simulink model "IdealGen_load_CtrlGen_wDC_abc"  (R2023b)
settings: Solver=VariableStepAuto  StartTime=0.0  StopTime=12  RelTol=1e-3
undefined symbols (not defined in the file): C_dc, H_vsm, I_dc_0, I_dc_base, Ibase_lv, k_d_vsm, k_p_p_vsm, k_p_q_vsm, ki_q, l_f, L_grid, Lbase1v, omega_nom, Pmax, r_f, R_grid, Sbase1, Tchange_gfm_ref, Ts, V_dc, V_dc_base, Vbase_lv, Zbase1v
libraries: spsControlledVoltageSourceLib x6, spsThreePhaseVIMeasurementLib x3, spsPower3phInstantaneousLib x3, spsRMSLib x3, spsdq0toabcLib x2, spsCurrentMeasurementLib x2, spsDCVoltageSourceLib x2, spsSeriesRLCBranchLib x2, spsVoltageMeasurementLib x2, slpidlib x2, spsThreePhaseSeriesRLCBranchLib x2, spsGroundLib x1
settings Model: Creator=s183702  LastModifiedBy=marti

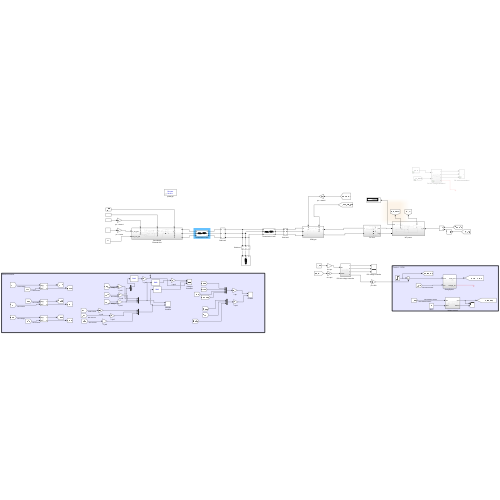
[thumbnail: Simulink's stored preview of the top-level diagram]
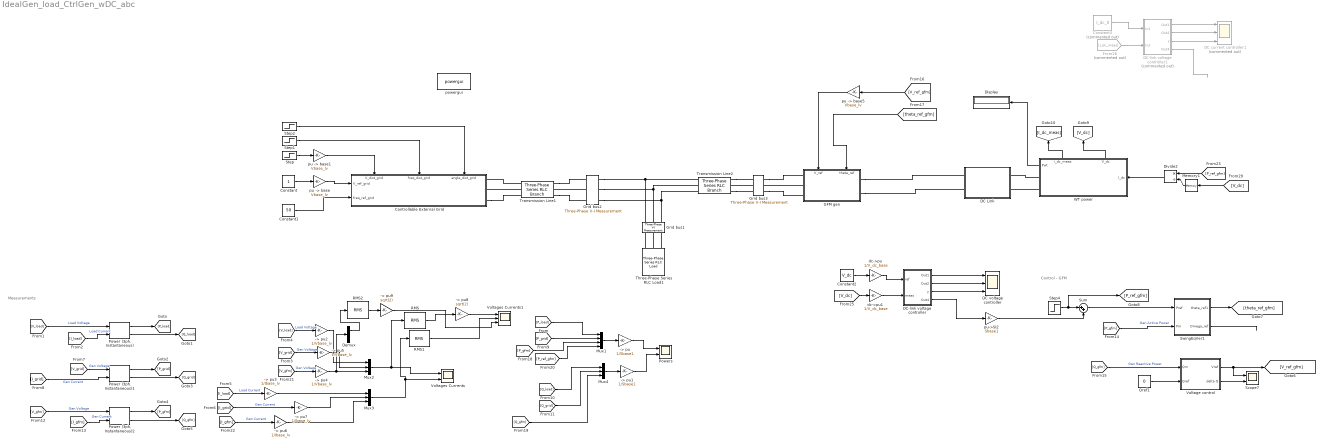
== system IdealGen_load_CtrlGen_wDC_abc ==
  note: Control - GFM
  note: Measurements
  -> pu : Gain  Gain=1/Sbase1
  -> pu1 : Gain  Gain=1/Sbase1
  -> pu2 : Gain  Gain=1/Vbase_lv
  -> pu3 : Gain  Gain=1/Ibase_lv
  -> pu4 : Gain  Gain=1/Vbase_lv
  -> pu5 : Gain  Gain=1/Vbase_lv
  -> pu6 : Gain  Gain=1/Ibase_lv
  -> pu7 : Gain  Gain=1/Ibase_lv
  -> pu8 : Gain  Gain=sqrt(2)
  -> pu9 : Gain  Gain=sqrt(2)
  Constant : Constant
  Constant1 : Constant  Value=50
  Constant2 : Constant  Value=V_dc
  Constant3 : Constant  Commented=on  Value=I_dc_0
  Controllable External Grid : Subsystem
      settings: PortSchema="{\"entries\":[{\"content\":{\"sides\":[{\"content\":{\"connectorIds\":[\"In1\",\"In2\"]},\"type\":\"ConnectorPlacement.EquallySpacedRectSide\",\"uuid\":\"c82e3ee4-47de-4631-9682-a189e406d2fd\"},{\"content\":{\"connectorIds\":[\"RConn1\",\"RConn2\",\"RConn3\"],\"side\":\"RIGHT\"},\"type\":\"ConnectorPlacement.EquallySpacedRectSide\",\"uuid\":\"b806e225-811d-4112-8c3d-45e9b8086e84\"},{\"content\":{\"connectorIds\":[\"In3\",\"In4\",\"In5\"],\"side\":\"TOP\"},\"type\":\"ConnectorPlacement.EquallySpacedRectSide\",\"uuid\":\"c79b677b-bc74-4454-b0f0-10f0f27e0767\"}]},\"type\":\"ConnectorPlacement.EquallySpacedConnector\",\"uuid\":\"44354c03-b4f0-403a-803b-b669dc1296a6\"}],\"packageUris\":[\"http://schema.mathworks.com/mf0/Connector/R2020b\"],\"version\":\"1.0\"}"
  DC Link : Subsystem
  DC current controller1 : Scope  Commented=on  NumInputPorts=3
  DC voltage controller : Scope  NumInputPorts=3
  DC-link voltage controller : Subsystem
  DC-link voltage controller1 : Subsystem  Commented=on
  Demux : Demux  Outputs=3
  Display : Display
  Divide2 : Product  Inputs=*/
  From26 : From  Commented=on  GotoTag=I_dc_meas
  GFM gen : Subsystem
      settings: PortSchema="{\"entries\":[{\"content\":{\"sides\":[{\"content\":{\"connectorIds\":[\"LConn1\",\"LConn2\"]},\"type\":\"ConnectorPlacement.EquallySpacedRectSide\",\"uuid\":\"b9b898d8-aa2c-4fc0-879f-33950e845205\"},{\"content\":{\"connectorIds\":[\"RConn1\",\"RConn2\",\"RConn3\"],\"side\":\"RIGHT\"},\"type\":\"ConnectorPlacement.EquallySpacedRectSide\",\"uuid\":\"0f5f2870-ceda-40eb-961f-274893a00dd5\"},{\"content\":{\"connectorIds\":[\"In1\",\"In2\"],\"side\":\"TOP\"},\"type\":\"ConnectorPlacement.EquallySpacedRectSide\",\"uuid\":\"16b0f3cd-2bcf-4c98-bcc9-1e9131637ccf\"}]},\"type\":\"ConnectorPlacement.EquallySpacedConnector\",\"uuid\":\"5f5ec50b-7fca-4ced-b434-e49ba9676af4\"}],\"packageUris\":[\"http://schema.mathworks.com/mf0/Connector/R2020b\"],\"version\":\"1.0\"}"
  Grid bus1 : spsThreePhaseVIMeasurementLib/Three-Phase V-I Measurement  VoltageMeasurement=phase-to-ground  SetLabelV=on  LabelV=V_load  Vpu=off  VpuLL=off  CurrentMeasurement=yes  SetLabelI=on  LabelI=I_load  Ipu=off  Pbase=100e6  Vbase=500e3  OutputType=Complex  PhasorSimulation=off  PSBequivalent=0
  Grid bus2 : spsThreePhaseVIMeasurementLib/Three-Phase V-I Measurement  VoltageMeasurement=phase-to-ground  SetLabelV=on  LabelV=V_grid  Vpu=off  VpuLL=off  CurrentMeasurement=yes  SetLabelI=on  LabelI=I_grid  Ipu=off  Pbase=100e6  Vbase=500e3  OutputType=Complex  PhasorSimulation=off  PSBequivalent=0
  Grid bus3 : spsThreePhaseVIMeasurementLib/Three-Phase V-I Measurement  VoltageMeasurement=phase-to-ground  SetLabelV=on  LabelV=V_gfm  Vpu=off  VpuLL=off  CurrentMeasurement=yes  SetLabelI=on  LabelI=I_gfm  Ipu=off  Pbase=100e6  Vbase=500e3  OutputType=Complex  PhasorSimulation=off  PSBequivalent=0
  Memory1 : Memory  InitialCondition=V_dc
  Mux1 : Mux
  Mux2 : Mux  Inputs=3
  Mux3 : Mux  Inputs=3
  Mux4 : Mux  Inputs=3
  "Power (3ph, Instantaneous)" : spsPower3phInstantaneousLib/Power (3ph, Instantaneous)
  "Power (3ph, Instantaneous)1" : spsPower3phInstantaneousLib/Power (3ph, Instantaneous)
  "Power (3ph, Instantaneous)2" : spsPower3phInstantaneousLib/Power (3ph, Instantaneous)
  Powers : Scope  NumInputPorts=2
  Qref1 : Constant  Value=0
  RMS : spsRMSLib/RMS  TrueRMS=on  Freq=50  RMSInit=1  Ts=0
  RMS1 : spsRMSLib/RMS  TrueRMS=on  Freq=50  RMSInit=1  Ts=0
  RMS2 : spsRMSLib/RMS  TrueRMS=on  Freq=50  RMSInit=1  Ts=0
  Scope7 : Scope  NumInputPorts=2
  Step : Step  After=0  SampleTime=0
  Step1 : Step  After=0  SampleTime=0
  Step2 : Step  After=0  SampleTime=0
  Step4 : Step  Time=Tchange_gfm_ref  Before=Sbase1  After=Sbase1  SampleTime=0
  Sum : Sum  Inputs=|++
  SwingEqVer1 : Subsystem
  Three-Phase Series RLC Load1 : spsThreePhaseSeriesRLCLoadLib/Three-Phase Series RLC Load  LConnTagsString=A|B|C  Configuration=Y (grounded)  NominalVoltage=Vbase_lv*sqrt(3/2)  Vabc=[1e3 1e3 1e3]  Vabcp=[1e3 1e3 1e3]  NominalFrequency=f_nom  UnbalancedPower=off  ActivePower=Sbase1*0.2  InductivePower=0  CapacitivePower=0  Pabc=[10e3 9e3 11e3]  QLabc=[100 90 110]  QCabc=[100 90 110]  Pabcp=[10e3 9e3 11e3]  QLabcp=[100 90 110]  QCabcp=[100 90 110]  Measurements=None  LoadType=constant PQ
  Transmission Line1 : spsThreePhaseSeriesRLCBranchLib/Three-Phase Series RLC Branch  LConnTagsString=A|B|C  RConnTagsString=A|B|C  BranchType=RL  Resistance=R_grid  Inductance=L_grid  Capacitance=0  Measurements=None
  Transmission Line2 : spsThreePhaseSeriesRLCBranchLib/Three-Phase Series RLC Branch  LConnTagsString=A|B|C  RConnTagsString=A|B|C  BranchType=RL  Resistance=r_f*Zbase1v  Inductance=l_f*Lbase1v  Capacitance=0  Measurements=None
  Voltage control : Subsystem
  Voltages Currents : Scope  NumInputPorts=2
  Voltages Currents1 : Scope  NumInputPorts=3
  WT power : Subsystem
      settings: PortSchema="{\"entries\":[{\"content\":{\"sides\":[{\"content\":{\"connectorIds\":[\"In1\"]},\"type\":\"ConnectorPlacement.EquallySpacedRectSide\",\"uuid\":\"9d3e38d2-6add-483d-9a31-3b5598dff8d3\"},{\"content\":{\"connectorIds\":[\"Out1\",\"RConn1\",\"RConn2\"],\"side\":\"RIGHT\"},\"type\":\"ConnectorPlacement.EquallySpacedRectSide\",\"uuid\":\"7ce5d226-07b0-4d85-bacd-eba224635451\"},{\"content\":{\"connectorIds\":[\"Out2\",\"Out3\"],\"side\":\"TOP\"},\"type\":\"ConnectorPlacement.EquallySpacedRectSide\",\"uuid\":\"1864accd-580c-4e01-b41e-4bc1921d0b77\"},{\"content\":{\"side\":\"BOTTOM\"},\"type\":\"ConnectorPlacement.EquallySpacedRectSide\",\"uuid\":\"0a771f6d-f5fb-412d-b2d7-9d95c39f39de\"}]},\"type\":\"ConnectorPlacement.EquallySpacedConnector\",\"uuid\":\"874bd654-abb7-47d1-80fe-1eaf36f4fe8a\"}],\"packageUris\":[\"http://schema.mathworks.com/mf0/Connector/R2020b\"],\"version\":\"1.0\"}"
  dc->pu : Gain  Gain=1/V_dc_base
  dc->pu1 : Gain  Gain=1/V_dc_base
  powergui : sps_lib/powergui  Priority=1  SimulationMode=Discrete  SampleTime=Ts  frequency=60  Iterations=50  frequencyindice=0  Pbase=100e6  ErrMax=1e-4  UnitsV=kV  UnitsW=MW  buscounter=0  FunctionMessages=off  echomessages=off  EnableUseOfTLC=off  CurrentSourceSwitches=off  DisableSnubberDevices=off  DisableRonSwitches=off  DisableVfSwitches=off  DisplayEquations=off  AutomaticDiscreteSolvers=off  SolverType=Tustin/Backward Euler (TBE)  Interpol=off  ExternalGateDelay=off  methode=off  Ts=100  x0status=blocks  SPID=on  SwTol=0  HookPort=off  NonlinearTolerance=1e-4  nMaxIteration=100  ContinueOnMaxIteration=off  RestoreLinks=warning  ResistiveCurrentMeasurement=off  Frange=[0:2:500]  Ylog=off  Xlog=on  ShowGrid=off  save=off  variable=ZData  structure=0  ZoomFFT=off  StartTime=0.0  cycles=1  DisplayStyle=1  fundamental=60  FreqAxis=off  MaxFrequency=1000  frequencyindicesteady=1  RmsSteady=1  display=off
  "pu -> base" : Gain  Gain=Vbase_lv
  "pu -> base1" : Gain  Gain=Vbase_lv
  "pu -> base5" : Gain  Gain=Vbase_lv
  pu->SI2 : Gain  Gain=Sbase1
  wires:
  [I_load] -> -> pu3/1  "Load Current"
  [V_load] -> -> pu2/1  "Load Voltage"
  [V_grid] -> -> pu5/1  "Gen Voltage"
  [I_grid] -> -> pu7/1  "Gen Current"
  "pu -> base"/1 -> Controllable External Grid/1(V_ref_grid)
  Constant/1 -> "pu -> base"/1
  Constant1/1 -> Controllable External Grid/2(freq_ref_grid)
  Step/1 -> "pu -> base1"/1
  Step1/1 -> Controllable External Grid/4(freq_dist_grid)
  Step2/1 -> Controllable External Grid/5(angle_dist_grid)
  "pu -> base1"/1 -> Controllable External Grid/3(V_dist_grid)
  [V_load] -> "Power (3ph, Instantaneous)"/1  "Load Voltage"
  [I_load] -> "Power (3ph, Instantaneous)"/2  "Load Current"
  [V_grid] -> "Power (3ph, Instantaneous)1"/1  "Gen Voltage"
  [I_grid] -> "Power (3ph, Instantaneous)1"/2  "Gen Current"
  "Power (3ph, Instantaneous)"/1 -> [P_load]
  "Power (3ph, Instantaneous)"/2 -> [Q_load]
  "Power (3ph, Instantaneous)1"/1 -> [P_grid]
  "Power (3ph, Instantaneous)1"/2 -> [Q_grid]
  [Q_load] -> Mux4/1
  [Q_grid] -> Mux4/2
  [P_grid] -> Mux1/2
  [P_load] -> Mux1/1
  Mux4/1 -> -> pu1/1
  Mux1/1 -> -> pu/1
  -> pu/1 -> Powers/1
  -> pu1/1 -> Powers/2
  "pu -> base5"/1 -> GFM gen/2(V_ref)
  "Power (3ph, Instantaneous)2"/2 -> [Q_gfm]
  "Power (3ph, Instantaneous)2"/1 -> [P_gfm]
  [I_gfm] -> "Power (3ph, Instantaneous)2"/2  "Gen Current"
  [V_gfm] -> "Power (3ph, Instantaneous)2"/1  "Gen Voltage"
  Sum/1 -> SwingEqVer1/1(Pref)
  [P_gfm] -> SwingEqVer1/2(Pm)  "Gen Active Power"
  SwingEqVer1/2(Omega_ref) -> ?
  SwingEqVer1/1(theta_ref1) -> [theta_ref_gfm]
  Qref1/1 -> Voltage control/2(Qref)
  Voltage control/1(Vref) -> Scope7/1, [V_ref_gfm]
  Voltage control/2(delta Q) -> Scope7/2
  [Q_gfm] -> Voltage control/1(Qm)  "Gen Reactive Power"
  [V_ref_gfm] -> "pu -> base5"/1
  [theta_ref_gfm] -> GFM gen/1(theta_ref)
  [P_gfm] -> Mux1/3
  [Q_gfm] -> Mux4/3
  [P_ref_gfm] -> Mux1/4
  [V_gfm] -> -> pu4/1  "Gen Voltage"
  [I_gfm] -> -> pu6/1  "Gen Current"
  Mux2/1 -> RMS/1, Voltages Currents/1
  Mux3/1 -> RMS1/1, Voltages Currents/2
  -> pu2/1 -> Mux2/1
  -> pu4/1 -> Demux/1, Mux2/3
  -> pu5/1 -> Mux2/2
  -> pu3/1 -> Mux3/1
  -> pu6/1 -> Mux3/3
  RMS/1 -> -> pu8/1
  RMS1/1 -> Voltages Currents1/2
  -> pu7/1 -> Mux3/2
  -> pu8/1 -> Voltages Currents1/1
  RMS2/1 -> -> pu9/1
  -> pu9/1 -> Voltages Currents1/3
  Demux/1 -> RMS2/1
  WT power/2(V_dc) -> [V_dc]
  WT power/1(Pwt) -> Display/1
  DC-link voltage controller1/4(Out4) -> ?
  Constant2/1 -> dc->pu/1
  [V_dc] -> dc->pu1/1
  DC-link voltage controller/1(Out1) -> DC voltage controller/1
  DC-link voltage controller/2(Out2) -> DC voltage controller/2
  DC-link voltage controller/3(y) -> DC voltage controller/3
  WT power/3(i_dc_meas) -> [I_dc_meas]
  From26/1 -> DC-link voltage controller1/2(In2)
  Constant3/1 -> DC-link voltage controller1/1(In1)
  DC-link voltage controller1/1(Out1) -> DC current controller1/1
  DC-link voltage controller1/2(Out2) -> DC current controller1/2
  DC-link voltage controller1/3(y) -> DC current controller1/3
  [P_ref_gfm] -> Divide2/1
  [V_dc] -> Memory1/1
  Memory1/1 -> Divide2/2
  Divide2/1 -> WT power/1(I_dc)
  dc->pu/1 -> DC-link voltage controller/1(ref)
  dc->pu1/1 -> DC-link voltage controller/2(meas)
  DC-link voltage controller/4(Out4) -> pu->SI2/1
  Step4/1 -> [P_ref_gfm], Sum/1
  pu->SI2/1 -> Sum/2
  connections:
  Three-Phase Series RLC Load1/LConn1 -- Grid bus1/RConn1
  Three-Phase Series RLC Load1/LConn2 -- Grid bus1/RConn2
  Three-Phase Series RLC Load1/LConn3 -- Grid bus1/RConn3
  Transmission Line2/LConn2 -- Grid bus2/RConn2 -- Grid bus1/LConn2
  Grid bus1/LConn1 -- Transmission Line2/LConn1 -- Grid bus2/RConn1
  Grid bus1/LConn3 -- Transmission Line2/LConn3 -- Grid bus2/RConn3
  Transmission Line1/RConn1 -- Grid bus2/LConn1
  Grid bus2/LConn2 -- Transmission Line1/RConn2
  Transmission Line1/RConn3 -- Grid bus2/LConn3
  Transmission Line1/LConn1 -- Controllable External Grid/RConn1
  Transmission Line1/LConn2 -- Controllable External Grid/RConn2
  Controllable External Grid/RConn3 -- Transmission Line1/LConn3
  GFM gen/RConn2 -- Grid bus3/LConn2
  Grid bus3/LConn1 -- GFM gen/RConn1
  Grid bus3/LConn3 -- GFM gen/RConn3
  Transmission Line2/RConn1 -- Grid bus3/RConn1
  Grid bus3/RConn2 -- Transmission Line2/RConn2
  Transmission Line2/RConn3 -- Grid bus3/RConn3
  GFM gen/LConn2 -- DC Link/LConn2
  GFM gen/LConn1 -- DC Link/LConn1
  WT power/RConn1 -- DC Link/RConn1
  WT power/RConn2 -- DC Link/RConn2

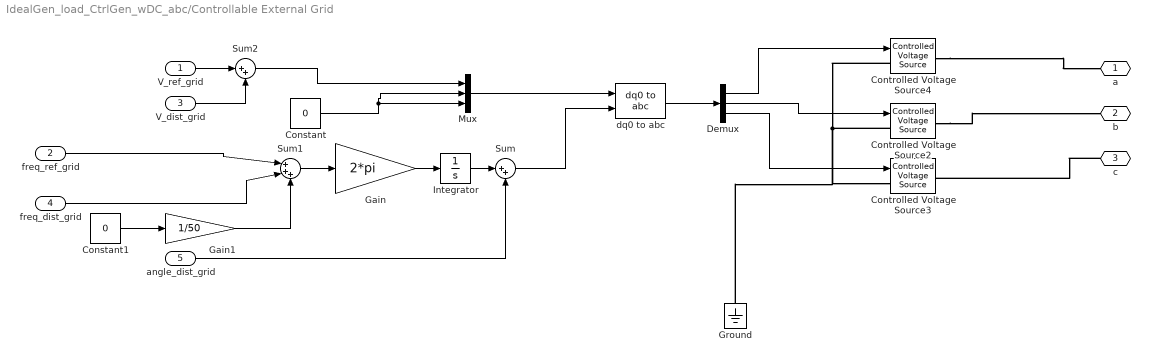
== system IdealGen_load_CtrlGen_wDC_abc/Controllable External Grid ==
  V_ref_grid : Inport
  freq_ref_grid : Inport  Port=2
  V_dist_grid : Inport  Port=3
  freq_dist_grid : Inport  Port=4
  angle_dist_grid : Inport  Port=5
  Constant : Constant  Value=0
  Constant1 : Constant  Value=0
  Controlled Voltage Source2 : spsControlledVoltageSourceLib/Controlled Voltage Source  Initialize=on  Source_Type=AC  Amplitude=Vbase_lv  Phase=-120  Frequency=50  Measurements=None
  Controlled Voltage Source3 : spsControlledVoltageSourceLib/Controlled Voltage Source  Initialize=on  Source_Type=AC  Amplitude=Vbase_lv  Phase=120  Frequency=50  Measurements=None
  Controlled Voltage Source4 : spsControlledVoltageSourceLib/Controlled Voltage Source  Initialize=on  Source_Type=AC  Amplitude=Vbase_lv  Phase=0  Frequency=50  Measurements=None
  Demux : Demux  Outputs=3
  Gain : Gain  Gain=2*pi
  Gain1 : Gain  Gain=1/50
  Ground : spsGroundLib/Ground  LConnTagsString=a
  Integrator : Integrator
  Mux : Mux  Inputs=3
  Sum : Sum  Inputs=|++
  Sum1 : Sum  Inputs=|+++
  Sum2 : Sum  Inputs=|++
  dq0 to abc : spsdq0toabcLib/dq0 to abc  Alignment=Aligned with phase A axis
  a : PMIOPort  Side=Right
  b : PMIOPort  Port=2  Side=Right
  c : PMIOPort  Port=3  Side=Right
  wires:
  Demux/1 -> Controlled Voltage Source4/1
  Demux/2 -> Controlled Voltage Source2/1
  Demux/3 -> Controlled Voltage Source3/1
  Mux/1 -> dq0 to abc/1
  Constant/1 -> Mux/2, Mux/3
  dq0 to abc/1 -> Demux/1
  Sum2/1 -> Mux/1
  Gain/1 -> Integrator/1
  Integrator/1 -> Sum/1
  angle_dist_grid/1 -> Sum/2
  freq_dist_grid/1 -> Sum1/2
  Sum1/1 -> Gain/1
  freq_ref_grid/1 -> Sum1/1
  Sum/1 -> dq0 to abc/2
  V_ref_grid/1 -> Sum2/1
  V_dist_grid/1 -> Sum2/2
  Gain1/1 -> Sum1/3
  Constant1/1 -> Gain1/1
  connections:
  Controlled Voltage Source2/LConn1 -- Controlled Voltage Source4/LConn1 -- Ground/LConn1 -- Controlled Voltage Source3/LConn1
  c/RConn1 -- Controlled Voltage Source3/RConn1
  Controlled Voltage Source4/RConn1 -- a/RConn1
  Controlled Voltage Source2/RConn1 -- b/RConn1

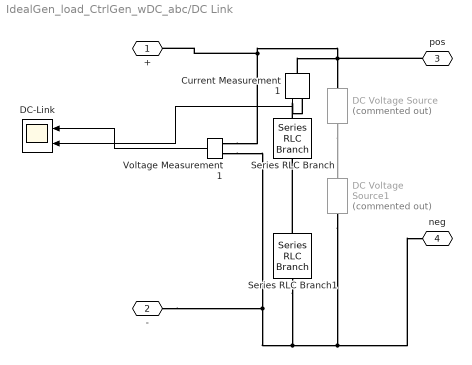
== system IdealGen_load_CtrlGen_wDC_abc/DC Link ==
  Current Measurement1 : spsCurrentMeasurementLib/Current Measurement  PhasorSimulation=off  OutputType=Complex  PSBequivalent=0
  DC Voltage Source : spsDCVoltageSourceLib/DC Voltage Source  Commented=on  Amplitude=V_dc/2  Measurements=None
  DC Voltage Source1 : spsDCVoltageSourceLib/DC Voltage Source  Commented=on  Amplitude=V_dc/2  Measurements=None
  DC-Link : Scope  NumInputPorts=2
  Series RLC Branch : spsSeriesRLCBranchLib/Series RLC Branch  LConnTagsString=__new0  RConnTagsString=__new0  BranchType=C  Resistance=1  Inductance=1e-3  SetiL0=off  InitialCurrent=0  Capacitance=C_dc/2  Setx0=on  InitialVoltage=V_dc/2  Measurements=None
  Series RLC Branch1 : spsSeriesRLCBranchLib/Series RLC Branch  LConnTagsString=__new0  RConnTagsString=__new0  BranchType=C  Resistance=1  Inductance=1e-3  SetiL0=off  InitialCurrent=0  Capacitance=C_dc/2  Setx0=on  InitialVoltage=V_dc/2  Measurements=None
  Voltage Measurement1 : spsVoltageMeasurementLib/Voltage Measurement  PhasorSimulation=off  OutputType=Complex  PSBequivalent=0
  + : PMIOPort  Side=Left
  - : PMIOPort  Port=2  Side=Left
  pos : PMIOPort  Port=3  Side=Right
  neg : PMIOPort  Port=4  Side=Right
  wires:
  Voltage Measurement1/1 -> DC-Link/1
  Current Measurement1/1 -> DC-Link/2
  connections:
  DC Voltage Source/LConn1 -- DC Voltage Source1/RConn1
  -/RConn1 -- Series RLC Branch1/RConn1 -- DC Voltage Source1/LConn1 -- neg/RConn1 -- Voltage Measurement1/LConn2
  Series RLC Branch1/LConn1 -- Series RLC Branch/RConn1
  pos/RConn1 -- Current Measurement1/LConn1 -- +/RConn1 -- Voltage Measurement1/LConn1 -- DC Voltage Source/RConn1
  Series RLC Branch/LConn1 -- Current Measurement1/RConn1

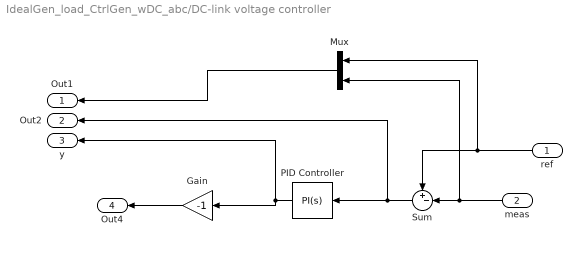
== system IdealGen_load_CtrlGen_wDC_abc/DC-link voltage controller ==
  ref : Inport
  meas : Inport  Port=2
  Gain : Gain  Gain=-1
  Mux : Mux  Inputs=2
  PID Controller : slpidlib/PID Controller  Controller=PI  Form=Parallel  TimeDomain=Continuous-time  UseExternalTs=off  SampleTime=-1  IntegratorMethod=Forward Euler  FilterMethod=Forward Euler  ControllerParametersSource=internal  P=5  I=1  UseKiTs=off  D=0  N=100  UseFilter=on  TunerSelectOption=Transfer Function Based (PID Tuner App)  InitialConditionSource=internal  InitialConditionForIntegrator=0  InitialConditionForFilter=0  DifferentiatorICPrevScaledInput=0  ExternalReset=none  TrackingMode=off  Kt=1  LimitOutput=off  SatLimitsSource=internal  UpperSaturationLimit=inf  LowerSaturationLimit=-inf  LinearizeAsGain=on  AntiWindupMode=none  Kb=1  LimitIntegrator=off  UpperIntegratorSaturationLimit=inf  LowerIntegratorSaturationLimit=-inf  POutMin=[]  POutMax=[]  IOutMin=[]  IOutMax=[]  DOutMin=[]  DOutMax=[]  NOutMin=[]  NOutMax=[]  SumOutMin=[]  SumOutMax=[]  SaturationOutMin=[]  SaturationOutMax=[]  PParamMin=[]  PParamMax=[]  IParamMin=[]  IParamMax=[]  DParamMin=[]  DParamMax=[]  NParamMin=[]  NParamMax=[]  KbParamMin=[]  KbParamMax=[]  KtParamMin=[]  KtParamMax=[]  KbOutMin=[]  KbOutMax=[]  KtOutMin=[]  KtOutMax=[]  IntegratorOutMin=[]  IntegratorOutMax=[]  FilterOutMin=[]  FilterOutMax=[]  SumI1OutMin=[]  SumI1OutMax=[]  SumI2OutMin=[]  SumI2OutMax=[]  SumI3OutMin=[]  SumI3OutMax=[]  SumI4OutMin=[]  SumI4OutMax=[]  SumDOutMin=[]  SumDOutMax=[]  DifferentiatorOutMin=[]  DifferentiatorOutMax=[]  FilterDiffOutCoefMin=[]  FilterDiffOutCoefMax=[]  ReciprocalOutMin=[]  ReciprocalOutMax=[]  SumDenOutMin=[]  SumDenOutMax=[]  SumNumOutMin=[]  SumNumOutMax=[]  DivideOutMin=[]  DivideOutMax=[]  UdiffTsProdOutMin=[]  UdiffTsProdOutMax=[]  NTsProdOutMin=[]  NTsProdOutMax=[]  UintegralTsProdOutMin=[]  UintegralTsProdOutMax=[]  UngainTsProdOutMin=[]  UngainTsProdOutMax=[]  ClampingZeroOutDataTypeStr=Inherit: Inherit via back propagation  ClampingZeroOutMin=[]  ClampingZeroOutMax=[]  FilterDenConstantOutDataTypeStr=Inherit: Inherit via back propagation  FilterDenConstantOutMin=[]  FilterDenConstantOutMax=[]  PCopyOutDataTypeStr=Inherit: Inherit via back propagation  PCopyOutMin=[]  PCopyOutMax=[]  NCopyOutDataTypeStr=Inherit: Inherit via back propagation  NCopyOutMin=[]  NCopyOutMax=[]  IntegratorContinuousStateAttributes=''  IntegratorStateMustResolveToSignalObject=off  IntegratorRTWStateStorageClass=Auto  FilterContinuousStateAttributes=''  FilterStateMustResolveToSignalObject=off  FilterRTWStateStorageClass=Auto  ParallelPVariant=InternalParameters  IdealPVariant=Disabled  IVariant=InternalParameters  DVariant=Disabled  IntegratorVariant=Continuous  SatVariant=Disabled  AWVariant=Passthrough  PCopyVariant=Disabled  TRVariant=Disabled  FdbkBlocksVariant=Forward  IdealPFdbkVariant=Disabled  SatFdbkVariant=Disabled  DerivativeFilterVariant=Disabled  NVariant=Disabled  NCopyVariant=Disabled_SignalSpec  FilterICVariant=Disabled  IntegratorICVariant=InternalICs  ExternalResetVariant=Disabled  TRSumVariant=Passthrough  SumFdbkVariant=Disabled  SumVariant=Sum_PI  TsampFilterVariant=InternalTs  TsampNgainVariant=Passthrough  TsampIntegralVariant=Disabled_SignalSpec  ExternalSaturationOutDataTypeStr=Inherit: Same as second input
  Sum : Sum  Inputs=+-|
  Out1 : Outport
  Out2 : Outport  Port=2
  y : Outport  Port=3
  Out4 : Outport  Port=4
  wires:
  Sum/1 -> Out2/1, PID Controller/1
  meas/1 -> Mux/2, Sum/2
  ref/1 -> Mux/1, Sum/1
  Mux/1 -> Out1/1
  PID Controller/1 -> y/1, Gain/1
  Gain/1 -> Out4/1

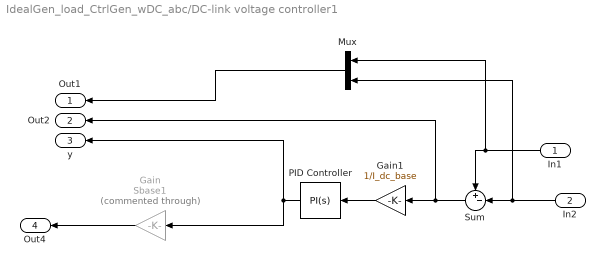
== system IdealGen_load_CtrlGen_wDC_abc/DC-link voltage controller1 ==
  In1 : Inport
  In2 : Inport  Port=2
  Gain : Gain  Commented=through  Gain=Sbase1
  Gain1 : Gain  Gain=1/I_dc_base
  Mux : Mux  Inputs=2
  PID Controller : slpidlib/PID Controller  Controller=PI  Form=Parallel  TimeDomain=Continuous-time  UseExternalTs=off  SampleTime=-1  IntegratorMethod=Forward Euler  FilterMethod=Forward Euler  ControllerParametersSource=internal  P=0.1  I=0  UseKiTs=off  D=0  N=100  UseFilter=on  TunerSelectOption=Transfer Function Based (PID Tuner App)  InitialConditionSource=internal  InitialConditionForIntegrator=1  InitialConditionForFilter=0  DifferentiatorICPrevScaledInput=0  ExternalReset=none  TrackingMode=off  Kt=1  LimitOutput=off  SatLimitsSource=internal  UpperSaturationLimit=inf  LowerSaturationLimit=-inf  LinearizeAsGain=on  AntiWindupMode=none  Kb=1  LimitIntegrator=off  UpperIntegratorSaturationLimit=inf  LowerIntegratorSaturationLimit=-inf  POutMin=[]  POutMax=[]  IOutMin=[]  IOutMax=[]  DOutMin=[]  DOutMax=[]  NOutMin=[]  NOutMax=[]  SumOutMin=[]  SumOutMax=[]  SaturationOutMin=[]  SaturationOutMax=[]  PParamMin=[]  PParamMax=[]  IParamMin=[]  IParamMax=[]  DParamMin=[]  DParamMax=[]  NParamMin=[]  NParamMax=[]  KbParamMin=[]  KbParamMax=[]  KtParamMin=[]  KtParamMax=[]  KbOutMin=[]  KbOutMax=[]  KtOutMin=[]  KtOutMax=[]  IntegratorOutMin=[]  IntegratorOutMax=[]  FilterOutMin=[]  FilterOutMax=[]  SumI1OutMin=[]  SumI1OutMax=[]  SumI2OutMin=[]  SumI2OutMax=[]  SumI3OutMin=[]  SumI3OutMax=[]  SumI4OutMin=[]  SumI4OutMax=[]  SumDOutMin=[]  SumDOutMax=[]  DifferentiatorOutMin=[]  DifferentiatorOutMax=[]  FilterDiffOutCoefMin=[]  FilterDiffOutCoefMax=[]  ReciprocalOutMin=[]  ReciprocalOutMax=[]  SumDenOutMin=[]  SumDenOutMax=[]  SumNumOutMin=[]  SumNumOutMax=[]  DivideOutMin=[]  DivideOutMax=[]  UdiffTsProdOutMin=[]  UdiffTsProdOutMax=[]  NTsProdOutMin=[]  NTsProdOutMax=[]  UintegralTsProdOutMin=[]  UintegralTsProdOutMax=[]  UngainTsProdOutMin=[]  UngainTsProdOutMax=[]  ClampingZeroOutDataTypeStr=Inherit: Inherit via back propagation  ClampingZeroOutMin=[]  ClampingZeroOutMax=[]  FilterDenConstantOutDataTypeStr=Inherit: Inherit via back propagation  FilterDenConstantOutMin=[]  FilterDenConstantOutMax=[]  PCopyOutDataTypeStr=Inherit: Inherit via back propagation  PCopyOutMin=[]  PCopyOutMax=[]  NCopyOutDataTypeStr=Inherit: Inherit via back propagation  NCopyOutMin=[]  NCopyOutMax=[]  IntegratorContinuousStateAttributes=''  IntegratorStateMustResolveToSignalObject=off  IntegratorRTWStateStorageClass=Auto  FilterContinuousStateAttributes=''  FilterStateMustResolveToSignalObject=off  FilterRTWStateStorageClass=Auto  ParallelPVariant=InternalParameters  IdealPVariant=Disabled  IVariant=InternalParameters  DVariant=Disabled  IntegratorVariant=Continuous  SatVariant=Disabled  AWVariant=Passthrough  PCopyVariant=Disabled  TRVariant=Disabled  FdbkBlocksVariant=Forward  IdealPFdbkVariant=Disabled  SatFdbkVariant=Disabled  DerivativeFilterVariant=Disabled  NVariant=Disabled  NCopyVariant=Disabled_SignalSpec  FilterICVariant=Disabled  IntegratorICVariant=InternalICs  ExternalResetVariant=Disabled  TRSumVariant=Passthrough  SumFdbkVariant=Disabled  SumVariant=Sum_PI  TsampFilterVariant=InternalTs  TsampNgainVariant=Passthrough  TsampIntegralVariant=Disabled_SignalSpec  ExternalSaturationOutDataTypeStr=Inherit: Same as second input
  Sum : Sum  Inputs=+-|
  Out1 : Outport
  Out2 : Outport  Port=2
  y : Outport  Port=3
  Out4 : Outport  Port=4
  wires:
  Gain/1 -> Out4/1
  PID Controller/1 -> Gain/1, y/1
  Mux/1 -> Out1/1
  In1/1 -> Sum/1, Mux/1
  In2/1 -> Sum/2, Mux/2
  Sum/1 -> Gain1/1, Out2/1
  Gain1/1 -> PID Controller/1

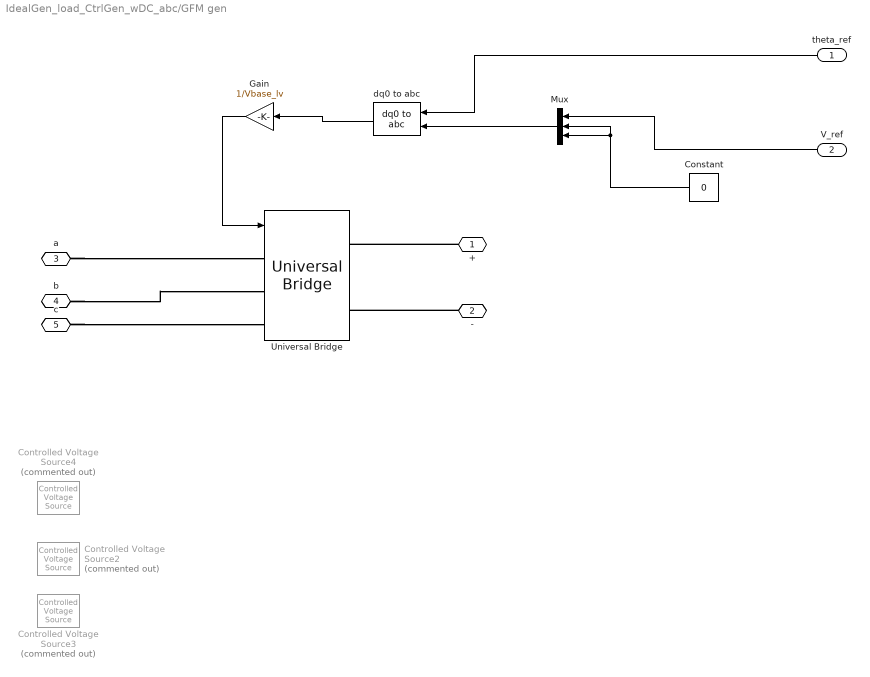
== system IdealGen_load_CtrlGen_wDC_abc/GFM gen ==
  theta_ref : Inport
  V_ref : Inport  Port=2
  Constant : Constant  Value=0
  Controlled Voltage Source2 : spsControlledVoltageSourceLib/Controlled Voltage Source  Commented=on  Initialize=on  Source_Type=AC  Amplitude=Vbase_lv  Phase=-120  Frequency=50  Measurements=None
  Controlled Voltage Source3 : spsControlledVoltageSourceLib/Controlled Voltage Source  Commented=on  Initialize=on  Source_Type=AC  Amplitude=Vbase_lv  Phase=120  Frequency=50  Measurements=None
  Controlled Voltage Source4 : spsControlledVoltageSourceLib/Controlled Voltage Source  Commented=on  Initialize=on  Source_Type=AC  Amplitude=Vbase_lv  Phase=0  Frequency=50  Measurements=None
  Gain : Gain  Gain=1/Vbase_lv
  Mux : Mux  Inputs=3
  Universal Bridge : spsUniversalBridgeLib/Universal Bridge  Arms=3  SnubberResistance=1e5  SnubberCapacitance=inf  Device=Average-model based VSC  Ron=1e-3  Lon=0  ForwardVoltages="[  0  0  ]"  ForwardVoltage=0  GTOparameters=[ 10e-6 , 20e-6 ]  IGBTparameters=[ 1e-6 , 2e-6 ]  Measurements=None  Measurements_2=None  converterType=Rectifier
  dq0 to abc : spsdq0toabcLib/dq0 to abc  Alignment=Aligned with phase A axis
  + : PMIOPort  Side=Left
  - : PMIOPort  Port=2  Side=Left
  a : PMIOPort  Port=3  Side=Right
  b : PMIOPort  Port=4  Side=Right
  c : PMIOPort  Port=5  Side=Right
  wires:
  Mux/1 -> dq0 to abc/1
  Constant/1 -> Mux/2, Mux/3
  dq0 to abc/1 -> Gain/1
  V_ref/1 -> Mux/1
  theta_ref/1 -> dq0 to abc/2
  Gain/1 -> Universal Bridge/1
  connections:
  c/RConn1 -- Universal Bridge/LConn3
  a/RConn1 -- Universal Bridge/LConn1
  b/RConn1 -- Universal Bridge/LConn2
  -/RConn1 -- Universal Bridge/RConn2
  +/RConn1 -- Universal Bridge/RConn1

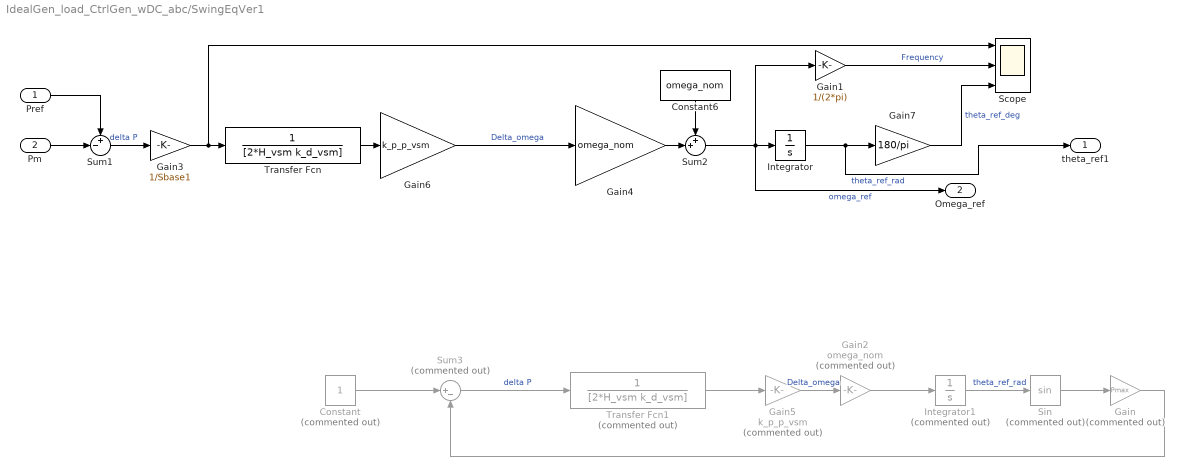
== system IdealGen_load_CtrlGen_wDC_abc/SwingEqVer1 ==
  Pref : Inport
  Pm : Inport  Port=2
  Constant : Constant  Commented=on
  Constant6 : Constant  Value=omega_nom
  Gain : Gain  Commented=on  Gain=Pmax
  Gain1 : Gain  Gain=1/(2*pi)
  Gain2 : Gain  Commented=on  Gain=omega_nom
  Gain3 : Gain  Gain=1/Sbase1
  Gain4 : Gain  Gain=omega_nom
  Gain5 : Gain  Commented=on  Gain=k_p_p_vsm
  Gain6 : Gain  Gain=k_p_p_vsm
  Gain7 : Gain  Gain=180/pi
  Integrator : Integrator  WrappedStateUpperValue=2*pi  WrappedStateLowerValue=0
  Integrator1 : Integrator  Commented=on  WrappedStateUpperValue=2*pi  WrappedStateLowerValue=0
  Scope : Scope  NumInputPorts=3
  Sin : Trigonometry  Commented=on
  Sum1 : Sum  Inputs=+-|
  Sum2 : Sum  Inputs=++|
  Sum3 : Sum  Commented=on  Inputs=|+-
  Transfer Fcn : TransferFcn  Denominator=[2*H_vsm k_d_vsm]
  Transfer Fcn1 : TransferFcn  Commented=on  Denominator=[2*H_vsm k_d_vsm]
  theta_ref1 : Outport
  Omega_ref : Outport  Port=2
  wires:
  Sum1/1 -> Gain3/1  "delta P"
  Integrator/1 -> theta_ref1/1, Gain7/1  "theta_ref_rad"
  Sum2/1 -> Gain1/1, Omega_ref/1, Integrator/1  "omega_ref"
  Transfer Fcn/1 -> Gain6/1
  Gain6/1 -> Gain4/1  "Delta_omega"
  Pm/1 -> Sum1/2
  Gain3/1 -> Scope/1, Transfer Fcn/1
  Gain7/1 -> Scope/3  "theta_ref_deg"
  Pref/1 -> Sum1/1
  Constant6/1 -> Sum2/1
  Gain4/1 -> Sum2/2
  Gain1/1 -> Scope/2  "Frequency"
  Gain5/1 -> Gain2/1  "Delta_omega"
  Transfer Fcn1/1 -> Gain5/1
  Sum3/1 -> Transfer Fcn1/1  "delta P"
  Gain2/1 -> Integrator1/1
  Sin/1 -> Gain/1
  Gain/1 -> Sum3/2
  Constant/1 -> Sum3/1
  Integrator1/1 -> Sin/1  "theta_ref_rad"

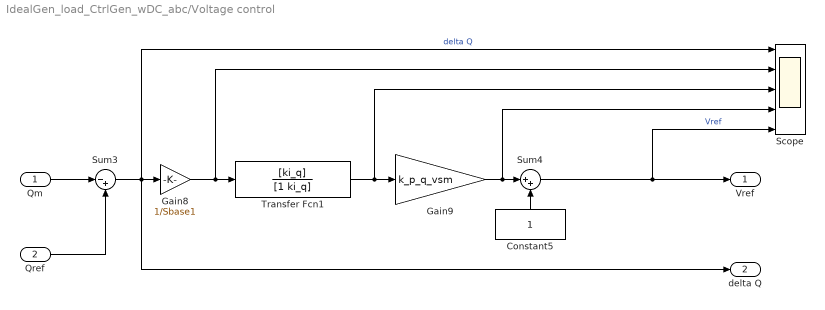
== system IdealGen_load_CtrlGen_wDC_abc/Voltage control ==
  Qm : Inport
  Qref : Inport  Port=2
  Constant5 : Constant
  Gain8 : Gain  Gain=1/Sbase1
  Gain9 : Gain  Gain=k_p_q_vsm
  Scope : Scope  NumInputPorts=5
  Sum3 : Sum  Inputs=|-+
  Sum4 : Sum  Inputs=|++
  Transfer Fcn1 : TransferFcn  Numerator=[ki_q]  Denominator=[1 ki_q]
  Vref : Outport
  delta Q : Outport  Port=2
  wires:
  Constant5/1 -> Sum4/2
  Qm/1 -> Sum3/1
  Gain9/1 -> Scope/4, Sum4/1
  Transfer Fcn1/1 -> Scope/3, Gain9/1
  Gain8/1 -> Scope/2, Transfer Fcn1/1
  Sum3/1 -> Scope/1, delta Q/1, Gain8/1  "delta Q"
  Sum4/1 -> Scope/5, Vref/1  "Vref"
  Qref/1 -> Sum3/2

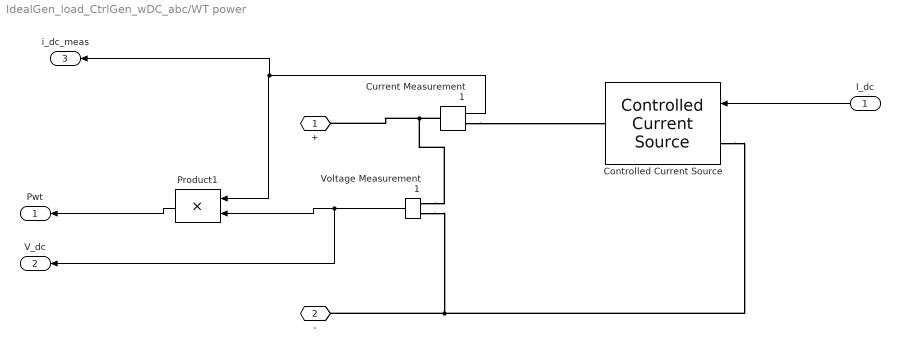
== system IdealGen_load_CtrlGen_wDC_abc/WT power ==
  I_dc : Inport
  Controlled Current Source : spsControlledCurrentSourceLib/Controlled Current Source  Initialize=on  Source_Type=DC  Amplitude=0  Phase=0  Frequency=0  Measurements=None
  Current Measurement1 : spsCurrentMeasurementLib/Current Measurement  PhasorSimulation=off  OutputType=Complex  PSBequivalent=0
  Product1 : Product  SaturateOnIntegerOverflow=on  OutDataTypeStr=Inherit: Same as first input
  Voltage Measurement1 : spsVoltageMeasurementLib/Voltage Measurement  PhasorSimulation=off  OutputType=Complex  PSBequivalent=0
  + : PMIOPort  Side=Right
  - : PMIOPort  Port=2  Side=Right
  Pwt : Outport
  V_dc : Outport  Port=2
  i_dc_meas : Outport  Port=3
  wires:
  Current Measurement1/1 -> i_dc_meas/1, Product1/1
  Product1/1 -> Pwt/1
  Voltage Measurement1/1 -> V_dc/1, Product1/2
  I_dc/1 -> Controlled Current Source/1
  connections:
  Controlled Current Source/LConn1 -- Voltage Measurement1/LConn2 -- -/RConn1
  Current Measurement1/LConn1 -- Voltage Measurement1/LConn1 -- +/RConn1
  Current Measurement1/RConn1 -- Controlled Current Source/RConn1
